simulink model "AirRefueling_Platform_PBVS_origin"  (R2022b)
settings: Solver=ode4  StartTime=0.0  StopTime=70  FixedStep=0.02  RelTol=1e-5  AbsTol=1e-4  EnableMultiTasking=on
InitFcn:
  | F16_Init
values from neighbouring files (symbols this model uses):
  airSpeed = 393.720000000000    (= 393.72)    [F16_Init.m]    (also in Initialization.m)
  alpha0 = trimAlpha*180/pi    (= 6.62393794015)    [F16_Init.m]    (also in Initialization.m)
  altitude = 9843    [F16_Init.m]    (also in Initialization.m)
  b_ref = 30.0    (= 30)    [F16_Init.m]    (also in Initialization.m)
  C = [ 1,0,0,zeros(1,15) ... (first row only)    [F16_Init.m]    (also in Initialization.m = [1,0,0,zeros(1,15))
  C2m = [C(1,:) ... (first row only)    [F16_Init.m]    (also in Initialization.m)
  d_f_rc = [3.75;0;-0.86]    [F16_Init.m]
  d_pr_rc = [6.06;0.54;-0.86]    [F16_Init.m]
  DeltaP = [0,0,DeltaP_z(j)]    [PBVS_main.m]
  dLEF = 0    [F16_Init.m]    (also in Initialization.m)
  fi_flag = 1    [F16_Init.m]    (also in Initialization.m)
  Kc = [ ... (first row only)    [F16_Init.m]    (also in Initialization.m)
  Ki = zeros(4,3)    [F16_Init.m]    (also in Initialization.m)
  Kp = zeros(4,18)    [F16_Init.m]    (also in Initialization.m)
  mass = 636.94    [F16_Init.m]    (also in Initialization.m)
  p0_rc = [-14.35-6.06-6;-0.54-(2);5.12+0.86-(-2)]    [F16_Init.m]
  q = zeros(N,1)    [hose3D_n_air_Fv_correction.m]
  trim_ail = 0.00874607850103852    (= 0.00874607850104)    [F16_Init.m]    (also in Initialization.m)
  trim_control = [trim_thrust;trim_ele;trim_ail;trim_rud]    [F16_Init.m]    (also in Initialization.m)
  trim_ele = -2.97973164860638    (= -2.97973164861)    [F16_Init.m]    (also in Initialization.m)
  trim_rud = 0.0680302158182712    (= 0.0680302158183)    [F16_Init.m]    (also in Initialization.m)
  trim_state1 = [trim_state;0;0;0;0;0;0]    [F16_Init.m]    (also in Initialization.m)
  trim_thrust = 2279.08519954656    (= 2279.08519955)    [F16_Init.m]    (also in Initialization.m)
undefined symbols (not defined in the file or in its folder): F, gray, MIL, vt0
libraries: aerolibconvert2 x6, aerolibasang x4, aerolibwind2 x2, aerolibobsolete x2, visionmorphops x2, vrlib x1, simulink x1, aerolibatmos2 x1, aerolibadyn x1, aerolibanimutils x1
(part 1 of 2)
settings Model: Creator=WhisPer  LastModifiedBy=Jinrui
settings SolverCC: AutoScaleAbsTol=off  AlgebraicLoopSolver=TrustRegion
settings DataIOCC: LimitDataPoints=on  SaveFormat=Array  ReturnWorkspaceOutputs=off
settings OptimizationCC: LifeSpan=inf
settings DebuggingCC: UnderspecifiedInitializationDetection=Classic  MergeDetectMultiDrivingBlocksExec=none  SolverPrmCheckMsg=warning  UnconnectedInputMsg=warning  UnconnectedOutputMsg=warning  UnconnectedLineMsg=warning  StateNameClashWarn=warning  SFUnexpectedBacktrackingDiag=warning  SFNoUnconditionalDefaultTransitionDiag=warning  SFExecutionAtInitializationDiag=none  SFMachineParentedDataDiag=warning  ArithmeticOperatorsInVariantConditions=warning
settings HardwareCC: ProdBitPerPointer=32  ProdBitPerSizeT=32  ProdBitPerPtrDiffT=32  ProdLargestAtomicFloat=None  ProdIntDivRoundTo=Undefined  ProdEndianess=Unspecified  ProdWordSize=32  ProdHWDeviceType=32-bit Generic
settings ModelReferenceCC: EnableRefExpFcnMdlSchedulingChecks=on  PropagateSignalLabelsOutOfModel=off
settings SFSimCC: SimUseLocalCustomCode=off  CustomCodeUndefinedFunction=UseInterfaceOnly
settings RTWCC: RTWUseLocalCustomCode=off
settings CodeAppCC: StateflowObjectComments=on
settings GRTTargetCC: TargetLangStandard=C89/C90 (ANSI)
settings ConfigComp: CovMetricSettings=dw  CovSaveCumulativeToWorkspaceVar=on  CovSaveSingleToWorkspaceVar=on  CovExternalEMLEnable=off

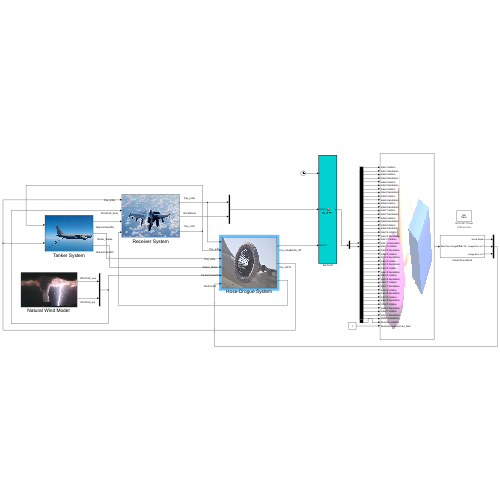
[thumbnail: Simulink's stored preview of the top-level diagram]
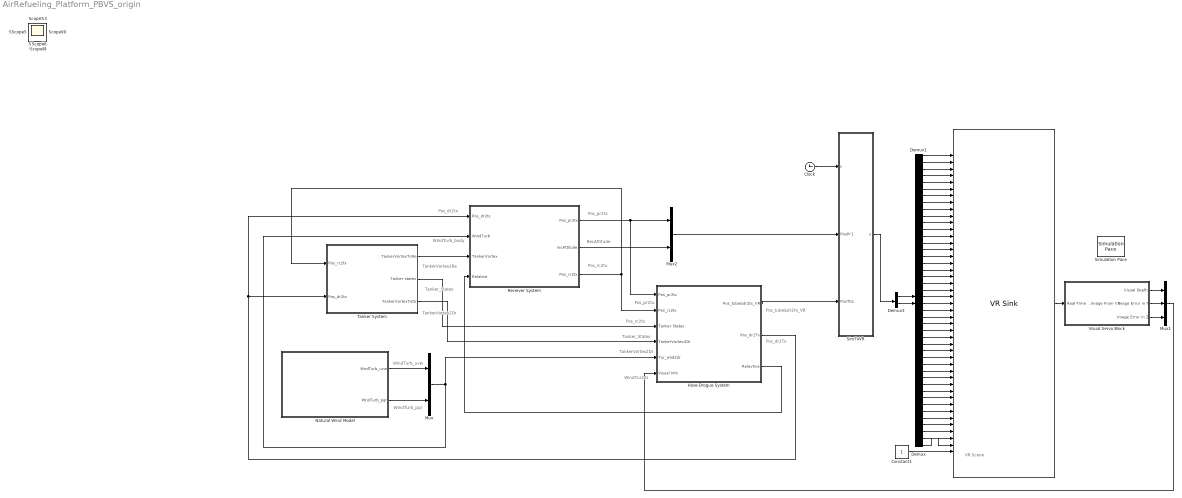
== system AirRefueling_Platform_PBVS_origin ==
  note: Pos_pr2tx
  note: RecAttitude
  note: WindTurb_uvw
  note: WindTurb_pqr
  note: Pos_dr2Tx
  note: Pos_tube&dr2tx_VR
  note: WindTur2dr
  note: Pos_pr2tx
  note: WindTurb_body
  note: Pos_dr2tx
  note: Pos_rc2tx
  note: TankerVortex2Re
  note: TankerVortex2Dr
  note: Tanker_States
  note: Tanker_States
  note: TankerVortex2Dr
  note: Pos_rc2tx
  note: VR Scene
  " " : vrlib/VR Sink  InstantiateOnLoad=on  SampleTime=-1  ViewEnable=on  RemoteChange=off  RemoteView=off  FieldsWritten=tube1.rotation.4.1.1.double#tube1.translation.3.1.1.double#tube2.rotation.4.1.1.double#tube2.translation.3.1.1.double#tube3.rotation.4.1.1.double#tube3.translation.3.1.1.double#tube4.rotation.4.1.1.double#tube4.translation.3.1.1.double#tube5.rotation.4.1.1.double#tube5.translation.3.1.1.double#tube6.rotation.4.1.1.double#tube6.translation.3.1.1.double#tube7.rotation.4.1.1.double#tube7.translation.3.1.1.double#tube8.rotation.4.1.1.double#tube8.translation.3.1.1.double#tube9.rotation.4.1.1.double#tube9.translation.3.1.1.double#tube10.rotation.4.1.1.double#tube10.translation.3.1.1.double#tube11.rotation.4.1.1.double#tube11.translation.3.1.1.double#tube12.rotation.4.1.1.double#tube12.translation.3.1.1.double#tube13.rotation.4.1.1.double#tube13.translation.3.1.1.double#tube14.rotation.4.1.1.double#tube14.translation.3.1.1.double#tube15.rotation.4.1.1.double#tube15.translation.3.1.1.double#tube16.rotation.4.1.1.double#tube16.translation.3.1.1.double#tube17.rotation.4.1.1.double#tube17.translation.3.1.1.double#tube18.rotation.4.1.1.double#tube18.translation.3.1.1.double#tube19.rotation.4.1.1.double#tube19.translation.3.1.1.double#tube20.rotation.4.1.1.double#tube20.translation.3.1.1.double#tube21.rotation.4.1.1.double#tube21.translation.3.1.1.double#ASDD.translation.3.1.1.double#Receiver.rotation.4.1.1.double#ReceiverViewPoint.set_bind.1.1.1.logical  WorldFileName=AirRefuelingTubeSim_Image.WRL  AutoView=off  VideoDimensions=[200 320]  AllowVariableSize=off  FigureProperties="{'Position', 'Name', 'Viewpoint', 'CameraBound', 'CameraDirection', 'CameraPosition', 'CameraUpVector', 'ZoomFactor', 'Antialiasing', 'Headlight', 'Lighting', 'NavPanel', 'Sound', 'StatusBar', 'Stereo3D', 'Stereo3DCameraOffset', 'Stereo3DHIT', 'ToolBar', 'Textures', 'Transparency', 'Triad', 'Wireframe', 'NavZones', 'NavMode', 'NavSpeed', 'CaptureFileFormat', 'CaptureFileName', 'Record2DCompressMethod', 'Record2DCompressQuality', 'Record2D', 'Record2DFileName', 'Record2DFPS'; [3.0000000000000000e+01   6.0000000000000000e+01   3.2000000000000000e+02   2.0000000000000000e+02], '', 'Receive1', 'on', [0.0000000000000000e+00   0.0000000000000000e+00  -1.0000000000000000e+00], [0.0000000000000000e+00   0.0000000000000000e+00   0.0000000000000000e+00], [0.0000000000000000e+00   1.0000000000000000e+00   0.0000000000000000e+00], [1.0000000000000000e+00], 'on', 'on', 'on', 'none', 'on', 'off', 'off', [1.0000000149011612e-01], [0.0000000000000000e+00], 'off', 'on', 'on', 'none', 'off', 'off', 'walk', 'normal', 'tif', '%f_anim_%n.tif', 'auto', [7.5000000000000000e+01], 'off', '***video***', 'auto'}"
  Clock : Clock
  Constant1 : Constant
  Demux : Demux  Outputs=22
  Demux1 : Demux  Outputs=22
  Demux3 : Demux  Outputs=[88,66]
  Hose-Drogue System : Subsystem
      mask Display: image(imread('Icon\drogue.jpg'))
  Mux : Mux  Inputs=2
  Mux1 : Mux  Inputs=3
  Mux2 : Mux  Inputs=2
  "Natural Wind Model " : Subsystem
      mask Display: image(imread('Icon\Enviroment.jpg'))
  Receiver System : Subsystem
      mask Display: image(imread('Icon\f16thumb.jpg'))
  SimToVR : MATLAB Function  TreatAsAtomicUnit=on
  Simulation Pace : aerolibanimutils/Simulation Pace  SimulationPace=1000  SleepMode=MATLAB Thread  OutputPaceError=off  SampleTime=-1
  Tanker System : Subsystem
      mask Display: image(imread('Icon\tanker.jpg'))
  Visual Servo Block : Subsystem
      mask Display: image('icon/camera.jpg');
  Scope{,1,3..34} (34 alike) : Scope
  wires:
  Receiver System/1(Pos_pr2tx) -> Hose-Drogue System/1(Pos_pr2tx), Mux2/1
  Hose-Drogue System/2(Pos_dr2Tx) -> Tanker System/2(Pos_dr2tx), Receiver System/1(Pos_dr2tx)
  Mux/1 -> Receiver System/2(WindTurb), Hose-Drogue System/5(Tur_wnd2dr)
  Receiver System/2(recAttitude) -> Mux2/2
  "Natural Wind Model "/1(WndTurb_uvw) -> Mux/1
  "Natural Wind Model "/2(WndTurb_pqr) -> Mux/2
  Tanker System/2(Tanker states) -> Hose-Drogue System/3(Tanker States)
  Tanker System/3(TankerVortexToDr) -> Hose-Drogue System/4(TankerVortex2Dr)
  Tanker System/1(TankerVortexToRe) -> Receiver System/3(TankerVortex)
  Receiver System/3(Pos_rc2tx) -> Hose-Drogue System/2(Pos_rc2tx), Tanker System/1(Pos_rc2tx)
  Hose-Drogue System/3(Relavtive) -> Receiver System/4(Relative)
  Hose-Drogue System/1(Pos_tube&dr2tx_VR) -> SimToVR/3(PosTb1)
  Mux2/1 -> SimToVR/2(PosPr1)
  Demux3/2 -> Demux/1
  Demux/22 -> " "/43
  Demux1/22 -> " "/44
  Demux3/1 -> Demux1/1
  Clock/1 -> SimToVR/1(t)
  Demux1/1 -> " "/1
  Demux/1 -> " "/2
  Demux1/2 -> " "/3
  Demux/2 -> " "/4
  Demux1/3 -> " "/5
  Demux/3 -> " "/6
  Demux1/4 -> " "/7
  Demux/4 -> " "/8
  Demux1/5 -> " "/9
  Demux/5 -> " "/10
  Demux1/6 -> " "/11
  Demux/6 -> " "/12
  Demux1/7 -> " "/13
  Demux/7 -> " "/14
  Demux1/8 -> " "/15
  Demux/8 -> " "/16
  Demux1/9 -> " "/17
  Demux/9 -> " "/18
  Demux1/10 -> " "/19
  Demux/10 -> " "/20
  Demux1/11 -> " "/21
  Demux/11 -> " "/22
  Demux1/12 -> " "/23
  Demux/12 -> " "/24
  Demux1/13 -> " "/25
  Demux/13 -> " "/26
  Demux1/14 -> " "/27
  Demux/14 -> " "/28
  Demux1/15 -> " "/29
  Demux/15 -> " "/30
  Demux1/16 -> " "/31
  Demux/16 -> " "/32
  Demux1/17 -> " "/33
  Demux/17 -> " "/34
  Demux1/18 -> " "/35
  Demux/18 -> " "/36
  Demux1/19 -> " "/37
  Demux/19 -> " "/38
  Demux1/20 -> " "/39
  Demux/20 -> " "/40
  Demux1/21 -> " "/41
  Demux/21 -> " "/42
  Constant1/1 -> " "/45
  " "/1 -> Visual Servo Block/1(Real-Time Image From VR)
  Visual Servo Block/1(Visual Depth) -> Mux1/1
  Visual Servo Block/2(Image Error in Y) -> Mux1/2
  Visual Servo Block/3(Image Error in Z) -> Mux1/3
  SimToVR/1(y) -> Demux3/1
  Mux1/1 -> Hose-Drogue System/6(Visual Info)

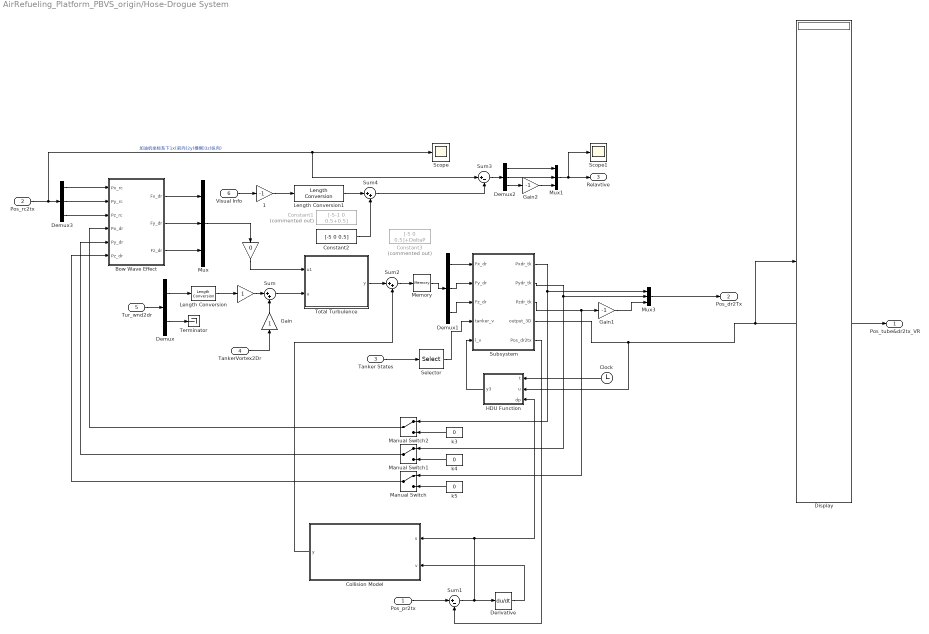
== system AirRefueling_Platform_PBVS_origin/Hose-Drogue System ==
  Pos_pr2tx : Inport
  Pos_rc2tx : Inport  Port=2
  Tanker States : Inport  Port=3
  TankerVortex2Dr : Inport  Port=4
  Tur_wnd2dr : Inport  Port=5
  Visual Info : Inport  Port=6
  " " : Gain
  "  " : Gain  Gain=0
  "  1" : Gain  Gain=-1
  Bow Wave Effect : Subsystem
  Clock : Clock
  Collision Model : MATLAB Function  TreatAsAtomicUnit=on
  Constant1 : Constant  Commented=on  Value=[-5-1 0 0.5+0.5]
  Constant2 : Constant  Value=[-5 0 0.5]
  Constant3 : Constant  Commented=on  Value=[-5 0 0.5]+DeltaP
  Demux : Demux  Outputs=2
  Demux1 : Demux  Outputs=3
  Demux2 : Demux  Outputs=3
  Demux3 : Demux  Outputs=3
  Derivative : Derivative
  Display : Display
  Gain : Gain
  Gain1 : Gain  Gain=-1
  Gain2 : Gain  Gain=-1
  HDU Function : MATLAB Function  TreatAsAtomicUnit=on
  Length Conversion : aerolibconvert2/Length Conversion  IU=ft  OU=m
  Length Conversion1 : aerolibconvert2/Length Conversion  IU=ft  OU=m
  Manual Switch : ManualSwitch
  Manual Switch1 : ManualSwitch
  Manual Switch2 : ManualSwitch
  Memory : Memory
  Mux : Mux  Inputs=3
  Mux1 : Mux  Inputs=3
  Mux3 : Mux  Inputs=3
  Scope : Scope
  Scope1 : Scope
  Selector : Selector  InputPortWidth=9  IndexOptions=Index vector (dialog)  Indices=[4 5 6]  OutputSizes=1
  Subsystem : Subsystem
  Sum : Sum  Inputs=|++
  Sum1 : Sum  Inputs=|+-
  Sum2 : Sum  Inputs=|++
  Sum3 : Sum  Inputs=|+-
  Sum4 : Sum  Inputs=|++
  Terminator : Terminator
  "Total Turbulence  " : MATLAB Function  TreatAsAtomicUnit=on
  k3 : Constant  Value=0
  k4 : Constant  Value=0
  k5 : Constant  Value=0
  Pos_tube&dr2tx_VR : Outport
  Pos_dr2Tx : Outport  Port=2
  Relavtive : Outport  Port=3
  wires:
  Mux/1 -> "  "/1
  TankerVortex2Dr/1 -> Gain/1
  Demux/1 -> Length Conversion/1
  Demux1/3 -> Subsystem/3(Fz_dr)
  Demux1/2 -> Subsystem/2(Fy_dr)
  Demux1/1 -> Subsystem/1(Fx_dr)
  Demux/2 -> Terminator/1
  Tur_wnd2dr/1 -> Demux/1
  Pos_rc2tx/1 -> Sum3/1, Scope/1, Demux3/1  "加油机坐标系下1x(前向)2y(横侧)3z(纵向)"
  Bow Wave Effect/3(Fz_dr) -> Mux/3
  Sum/1 -> "Total Turbulence  "/2(u)
  Bow Wave Effect/2(Fy_dr) -> Mux/2
  Bow Wave Effect/1(Fx_dr) -> Mux/1
  Demux3/1 -> Bow Wave Effect/1(Px_rc)
  k4/1 -> Manual Switch1/2
  Manual Switch1/1 -> Bow Wave Effect/5(Py_dr)
  Manual Switch2/1 -> Bow Wave Effect/4(Px_dr)
  k5/1 -> Manual Switch/2
  k3/1 -> Manual Switch2/2
  Mux3/1 -> Pos_dr2Tx/1
  Manual Switch/1 -> Bow Wave Effect/6(Pz_dr)
  Subsystem/2(Pydr_tk) -> Manual Switch1/1, Mux3/2
  Subsystem/1(Pxdr_tk) -> Manual Switch2/1, Mux3/1
  Gain1/1 -> Mux3/3
  Subsystem/3(Pzdr_tk) -> Gain1/1, Manual Switch/1
  Demux3/3 -> Bow Wave Effect/3(Pz_rc)
  Demux3/2 -> Bow Wave Effect/2(Py_rc)
  "Total Turbulence  "/1(y) -> Sum2/1
  Subsystem/4(output_3D) -> Display/1, Pos_tube&dr2tx_VR/1, HDU Function/2(u)
  Gain/1 -> Sum/2
  " "/1 -> Sum/1
  "  "/1 -> "Total Turbulence  "/1(u1)
  Length Conversion/1 -> " "/1
  Tanker States/1 -> Selector/1
  Sum1/1 -> Collision Model/1(u), HDU Function/3(dp), Derivative/1
  Derivative/1 -> Collision Model/2(v)
  Sum2/1 -> Memory/1
  Selector/1 -> Subsystem/4(tanker_v)
  Subsystem/5(Pos_dr2tx) -> Sum1/2
  Memory/1 -> Demux1/1
  Clock/1 -> HDU Function/1(t)
  HDU Function/1(y3) -> Subsystem/5(l_v)
  Pos_pr2tx/1 -> Sum1/1
  Visual Info/1 -> "  1"/1
  "  1"/1 -> Length Conversion1/1
  Length Conversion1/1 -> Sum4/1
  Sum4/1 -> Sum3/2
  Constant2/1 -> Sum4/2
  Demux2/2 -> Mux1/2
  Demux2/1 -> Mux1/1
  Gain2/1 -> Mux1/3
  Demux2/3 -> Gain2/1
  Mux1/1 -> Relavtive/1, Scope1/1
  Sum3/1 -> Demux2/1
  Collision Model/1(y) -> Sum2/2

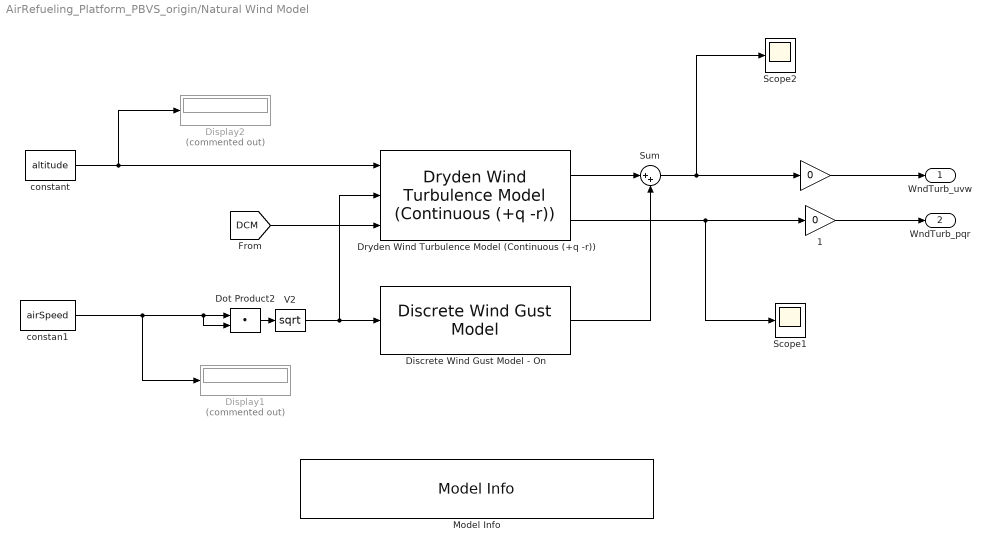
== system AirRefueling_Platform_PBVS_origin/Natural Wind Model  ==
  " " : Gain  Gain=0
  " 1" : Gain  Gain=0
  Discrete Wind Gust Model - On : aerolibwind2/Discrete Wind Gust Model  units=English (Velocity in ft/s)  Gx=on  Gy=on  Gz=on  t_0=20  d_m=[120 120 80]  v_m=[0 0 0]
  Display1 : Display  Commented=on
  Display2 : Display  Commented=on
  Dot Product2 : DotProduct  SaturateOnIntegerOverflow=on  InputSameDT=off  OutDataTypeStr=Inherit: Inherit via internal rule
  Dryden Wind Turbulence Model (Continuous (+q -r)) : aerolibwind2/Dryden Wind Turbulence Model  (Continuous (+q -r))  units=English (Velocity in ft/s)  spec=MIL-F-8785C  model=Continuous Dryden (+q -r)  W20=5  Wdeg=0  TurbProb=2x10^-1  L_high=533.5  Wingspan=6  ts=0.02  Seed=1+fix(3650*rand(1,4))  T_on=on
  Model Info : simulink/Model-Wide Utilities/Model Info  Frame=on  DisplayStringWithTags=|  HorizontalTextAlignment=Center  LeftAlignmentValue=0.5
      | The resultant mean wind speed and angular rates is in the body-fixed axis. 
      | The simulation parameter is set to
      | altitude:3000m
      | airspeed:120m/s
  Scope1 : Scope
  Scope2 : Scope
  Sum : Sum  Inputs=|++  InputSameDT=on  SaturateOnIntegerOverflow=on  OutDataTypeStr=Inherit: Same as first input
  V2 : Math  Operator=sqrt  SignedPower=on
  constan1 : Constant  Value=airSpeed
  constant : Constant  Value=altitude
  WndTurb_uvw : Outport
  WndTurb_pqr : Outport  Port=2
  wires:
  [DCM] -> Dryden Wind Turbulence Model (Continuous (+q -r))/3
  V2/1 -> Dryden Wind Turbulence Model (Continuous (+q -r))/2, Discrete Wind Gust Model - On/1
  Dot Product2/1 -> V2/1
  constan1/1 -> Dot Product2/1, Dot Product2/2, Display1/1
  Discrete Wind Gust Model - On/1 -> Sum/2
  Dryden Wind Turbulence Model (Continuous (+q -r))/2 -> Scope1/1, " 1"/1
  Dryden Wind Turbulence Model (Continuous (+q -r))/1 -> Sum/1
  Sum/1 -> Scope2/1, " "/1
  constant/1 -> Display2/1, Dryden Wind Turbulence Model (Continuous (+q -r))/1
  " "/1 -> WndTurb_uvw/1
  " 1"/1 -> WndTurb_pqr/1

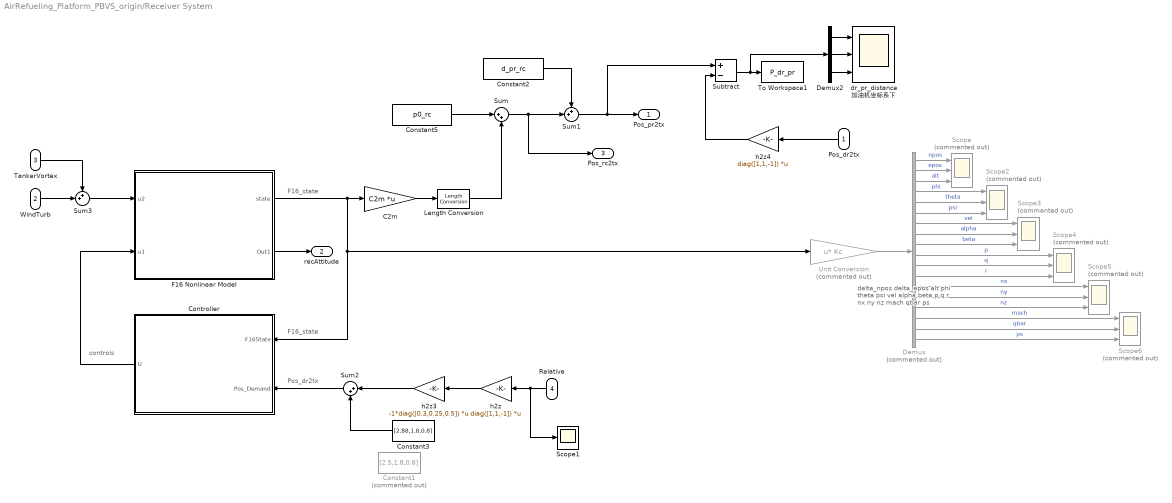
== system AirRefueling_Platform_PBVS_origin/Receiver System ==
  note: controls
  note: Pos_dr2tx
  note: F16_state
  note: delta_npos
      | delta_epos
      | alt
      | phi
      | theta
      | psi
      | vel
      | alpha
      | beta
      | p
      | q
      | r
      | nx
      | ny
      | nz
      | mach
      | qbar
      | ps
  note: F16_state
  Pos_dr2tx : Inport
  WindTurb : Inport  Port=2
  TankerVortex : Inport  Port=3
  Relative : Inport  Port=4
  C2m : Gain  Gain=C2m  Multiplication=Matrix(K*u) (u vector)
  Constant1 : Constant  Commented=on  Value=[2.5,1.8,0.8]
  Constant2 : Constant  Value=d_pr_rc
  Constant3 : Constant  Value=[2.88,1.8,0.8]
  Constant5 : Constant  Value=p0_rc
  Controller : Subsystem
      mask Display: image(imread('Icon\F16_Pilot.jpg'))
  Demux : Demux  Commented=on  Outputs=18
      settings: DisplayOption=none
  Demux2 : Demux  Outputs=3
  F16 Nonlinear Model : Subsystem
      mask Display: image(imread('Icon\fighter_f16.jpg'))
  Length Conversion : aerolibconvert2/Length Conversion  IU=ft  OU=m
  Scope{,2..6} (6 alike) : Scope  Commented=on  NumInputPorts=3
  Scope1 : Scope
  Subtract : Sum  Inputs=+-
  Sum : Sum  Inputs=|++
  Sum1 : Sum  Inputs=++|
  Sum2 : Sum  Inputs=|++
  Sum3 : Sum  Inputs=++|
  To Workspace1 : ToWorkspace  VariableName=P_dr_pr  SampleTime=-1
  Unit Conversion : Gain  Commented=on  Gain=Kc  Multiplication=Matrix(u*K)
  dr_pr_distance 加油机坐标系下 : Scope  NumInputPorts=3
  h2z : Gain  Gain=diag([1,1,-1])  Multiplication=Matrix(K*u)
  h2z3 : Gain  Gain=-1*diag([0.3,0.25,0.5])  Multiplication=Matrix(K*u)
  h2z4 : Gain  Gain=diag([1,1,-1])  Multiplication=Matrix(K*u)
  Pos_pr2tx : Outport
  recAttitude : Outport  Port=2
  Pos_rc2tx : Outport  Port=3
  wires:
  Controller/1(U) -> F16 Nonlinear Model/2(u1)
  WindTurb/1 -> Sum3/2
  F16 Nonlinear Model/1(state) -> C2m/1, Controller/1(F16State), Unit Conversion/1
  Demux/1 -> Scope/1  "npos"
  Demux/2 -> Scope/2  "epos"
  Demux/3 -> Scope/3  "alt"
  Demux/5 -> Scope2/2  "theta"
  Demux/6 -> Scope2/3  "psi"
  Demux/7 -> Scope3/1  "vel"
  Demux/8 -> Scope3/2  "alpha"
  Demux/9 -> Scope3/3  "beta"
  Demux/10 -> Scope4/1  "p"
  Demux/11 -> Scope4/2  "q"
  Demux/12 -> Scope4/3  "r"
  Demux/13 -> Scope5/1  "nx"
  Demux/14 -> Scope5/2  "ny"
  Demux/15 -> Scope5/3  "nz"
  Demux/4 -> Scope2/1  "phi"
  Demux/16 -> Scope6/1  "mach"
  Demux/17 -> Scope6/2  "qbar"
  Demux/18 -> Scope6/3  "ps"
  Unit Conversion/1 -> Demux/1
  F16 Nonlinear Model/2(Out1) -> recAttitude/1
  C2m/1 -> Length Conversion/1
  Sum3/1 -> F16 Nonlinear Model/1(u2)
  TankerVortex/1 -> Sum3/1
  Length Conversion/1 -> Sum/2
  Constant5/1 -> Sum/1
  Sum1/1 -> Pos_pr2tx/1, Subtract/1
  Sum/1 -> Pos_rc2tx/1, Sum1/2
  Constant2/1 -> Sum1/1
  h2z/1 -> h2z3/1
  Sum2/1 -> Controller/2(Pos_Demand)
  h2z3/1 -> Sum2/1
  Constant3/1 -> Sum2/2
  Pos_dr2tx/1 -> h2z4/1
  Subtract/1 -> Demux2/1, To Workspace1/1
  Demux2/2 -> dr_pr_distance 加油机坐标系下/2
  Demux2/1 -> dr_pr_distance 加油机坐标系下/1
  Demux2/3 -> dr_pr_distance 加油机坐标系下/3
  h2z4/1 -> Subtract/2
  Relative/1 -> Scope1/1, h2z/1

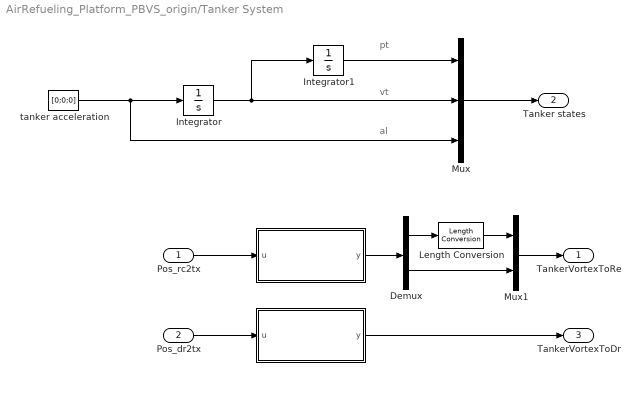
== system AirRefueling_Platform_PBVS_origin/Tanker System ==
  note: pt
  note: vt
  note: al
  Pos_rc2tx : Inport
  Pos_dr2tx : Inport  Port=2
  " " : MATLAB Function  TreatAsAtomicUnit=on
  "  " : MATLAB Function  TreatAsAtomicUnit=on
  Demux : Demux  Outputs=2
  Integrator : Integrator  InitialCondition=vt0
  Integrator1 : Integrator  InitialCondition=[0;0;0]
  Length Conversion : aerolibconvert2/Length Conversion  IU=m  OU=ft
  Mux : Mux  Inputs=3
  Mux1 : Mux  Inputs=2
  tanker acceleration : Constant  Value=[0;0;0]
  TankerVortexToRe : Outport
  Tanker states : Outport  Port=2
  TankerVortexToDr : Outport  Port=3
  wires:
  tanker acceleration/1 -> Mux/3, Integrator/1
  Integrator/1 -> Mux/2, Integrator1/1
  Mux/1 -> Tanker states/1
  Pos_rc2tx/1 -> " "/1(u)
  Pos_dr2tx/1 -> "  "/1(u)
  "  "/1(y) -> TankerVortexToDr/1
  Integrator1/1 -> Mux/1
  " "/1(y) -> Demux/1
  Mux1/1 -> TankerVortexToRe/1
  Demux/2 -> Mux1/2
  Length Conversion/1 -> Mux1/1
  Demux/1 -> Length Conversion/1

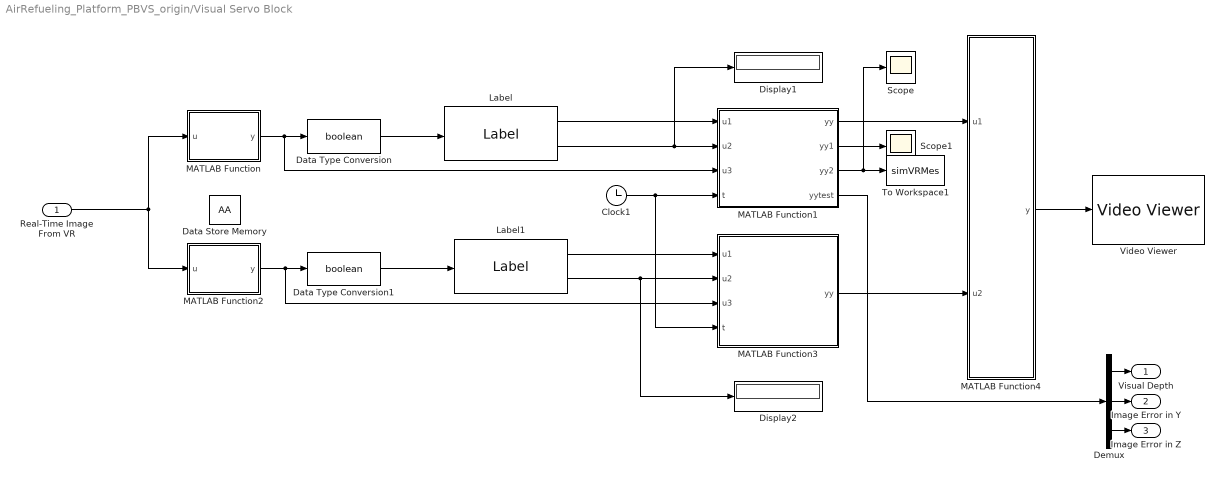
== system AirRefueling_Platform_PBVS_origin/Visual Servo Block ==
  Real-Time Image From VR : Inport
  Clock1 : Clock
  Data Store Memory : DataStoreMemory  DataStoreName=AA  InitialValue=[0 0 0]  ShowAdditionalParam=off  OutDataTypeStr=double
  Data Type Conversion : DataTypeConversion  OutDataTypeStr=boolean  SaturateOnIntegerOverflow=off  RndMeth=Floor
  Data Type Conversion1 : DataTypeConversion  OutDataTypeStr=boolean  SaturateOnIntegerOverflow=off  RndMeth=Floor
  Demux : Demux  Outputs=3
  Display1 : Display
  Display2 : Display
  Label : visionmorphops/Label  conn=8  output=Label matrix and number of labels  outType=Automatic  lastLabel=maximum value of the output data type
  Label1 : visionmorphops/Label  conn=8  output=Label matrix and number of labels  outType=Automatic  lastLabel=maximum value of the output data type
  MATLAB Function : MATLAB Function  TreatAsAtomicUnit=on
  MATLAB Function1 : MATLAB Function  TreatAsAtomicUnit=on
  MATLAB Function2 : MATLAB Function  TreatAsAtomicUnit=on
  MATLAB Function3 : MATLAB Function  TreatAsAtomicUnit=on
  MATLAB Function4 : MATLAB Function  TreatAsAtomicUnit=on
  Scope : Scope
  Scope1 : Scope
  To Workspace1 : ToWorkspace  VariableName=simVRMes  SampleTime=-1
  Video Viewer : VideoViewer  colormapValue=gray(256)  FigPos=[840 825 710 515]
  Visual Depth : Outport
  Image Error in Y : Outport  Port=2
  Image Error in Z : Outport  Port=3
  wires:
  Real-Time Image From VR/1 -> MATLAB Function/1(u), MATLAB Function2/1(u)
  Label/1 -> MATLAB Function1/1(u1)
  MATLAB Function/1(y) -> MATLAB Function1/3(u3), Data Type Conversion/1
  Data Type Conversion/1 -> Label/1
  MATLAB Function2/1(y) -> MATLAB Function3/3(u3), Data Type Conversion1/1
  Data Type Conversion1/1 -> Label1/1
  Label1/1 -> MATLAB Function3/1(u1)
  Label1/2 -> Display2/1, MATLAB Function3/2(u2)
  MATLAB Function1/1(yy) -> MATLAB Function4/1(u1)
  MATLAB Function3/1(yy) -> MATLAB Function4/2(u2)
  MATLAB Function4/1(y) -> Video Viewer/1
  Clock1/1 -> MATLAB Function3/4(t), MATLAB Function1/4(t)
  Label/2 -> Display1/1, MATLAB Function1/2(u2)
  MATLAB Function1/4(yytest) -> Demux/1
  Demux/1 -> Visual Depth/1
  Demux/2 -> Image Error in Y/1
  Demux/3 -> Image Error in Z/1
  MATLAB Function1/3(yy2) -> Scope/1, To Workspace1/1
  MATLAB Function1/2(yy1) -> Scope1/1

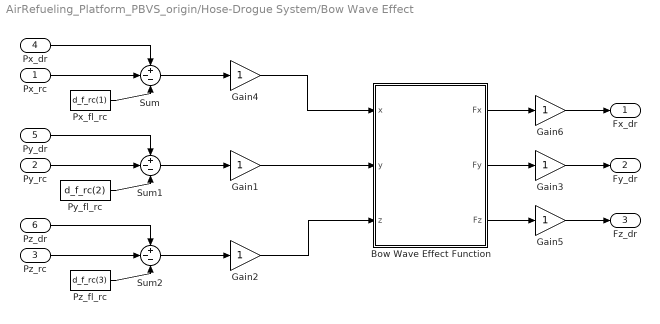
== system AirRefueling_Platform_PBVS_origin/Hose-Drogue System/Bow Wave Effect ==
  Px_rc : Inport
  Py_rc : Inport  Port=2
  Pz_rc : Inport  Port=3
  Px_dr : Inport  Port=4
  Py_dr : Inport  Port=5
  Pz_dr : Inport  Port=6
  Bow Wave Effect Function : MATLAB Function  TreatAsAtomicUnit=on
  Gain{1..6} (6 alike) : Gain
  Px_fl_rc : Constant  Value=d_f_rc(1)
  Py_fl_rc : Constant  Value=d_f_rc(2)
  Pz_fl_rc : Constant  Value=d_f_rc(3)
  Sum : Sum  Inputs=+--
  Sum1 : Sum  Inputs=+--
  Sum2 : Sum  Inputs=+--
  Fx_dr : Outport
  Fy_dr : Outport  Port=2
  Fz_dr : Outport  Port=3
  wires:
  Sum2/1 -> Gain2/1
  Sum1/1 -> Gain1/1
  Bow Wave Effect Function/3(Fz) -> Gain5/1
  Bow Wave Effect Function/2(Fy) -> Gain3/1
  Bow Wave Effect Function/1(Fx) -> Gain6/1
  Gain6/1 -> Fx_dr/1
  Gain5/1 -> Fz_dr/1
  Gain3/1 -> Fy_dr/1
  Gain2/1 -> Bow Wave Effect Function/3(z)
  Gain1/1 -> Bow Wave Effect Function/2(y)
  Gain4/1 -> Bow Wave Effect Function/1(x)
  Pz_dr/1 -> Sum2/1
  Pz_fl_rc/1 -> Sum2/3
  Pz_rc/1 -> Sum2/2
  Py_fl_rc/1 -> Sum1/3
  Py_dr/1 -> Sum1/1
  Py_rc/1 -> Sum1/2
  Px_dr/1 -> Sum/1
  Px_fl_rc/1 -> Sum/3
  Px_rc/1 -> Sum/2
  Sum/1 -> Gain4/1

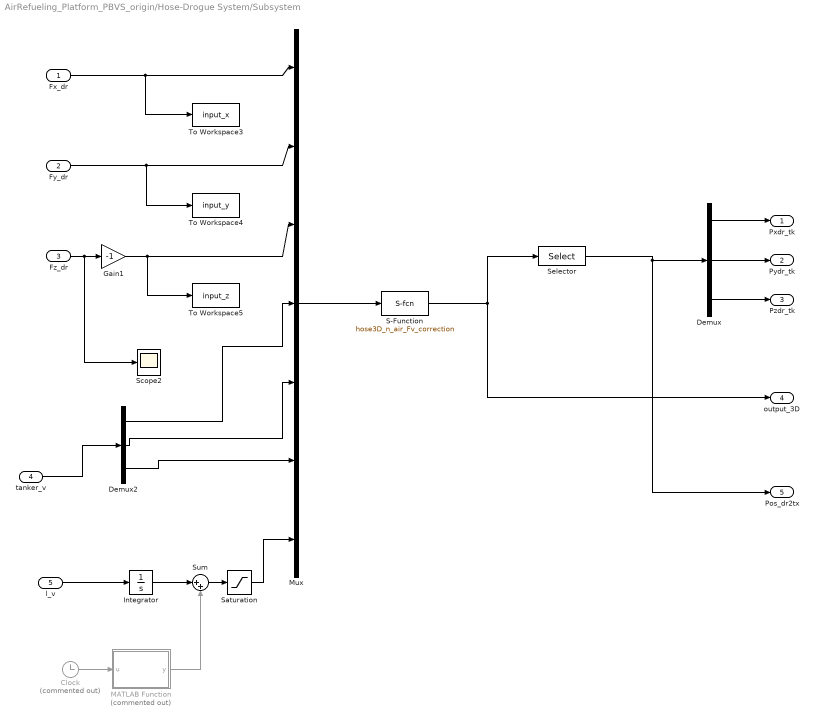
== system AirRefueling_Platform_PBVS_origin/Hose-Drogue System/Subsystem ==
  Fx_dr : Inport
  Fy_dr : Inport  Port=2
  Fz_dr : Inport  Port=3
  tanker_v : Inport  Port=4
  l_v : Inport  Port=5
  Clock : Clock  Commented=on
  Demux : Demux  Outputs=3
  Demux2 : Demux  Outputs=3
  Gain1 : Gain  Gain=-1  ParamDataTypeStr=double  OutDataTypeStr=double
  Integrator : Integrator
  MATLAB Function : MATLAB Function  Commented=on  TreatAsAtomicUnit=on
  Mux : Mux  Inputs=7
  S-Function : S-Function  FunctionName=hose3D_n_air_Fv_correction  SFunctionDeploymentMode=off  EnableBusSupport=off
  Saturation : Saturate  UpperLimit=13  LowerLimit=-1
  Scope2 : Scope
  Selector : Selector  InputPortWidth=100  IndexOptions=Index vector (dialog)  Indices=[58 59 60]  OutputSizes=1
  Sum : Sum  Inputs=|++
  To Workspace3 : ToWorkspace  VariableName=input_x  SampleTime=-1
  To Workspace4 : ToWorkspace  VariableName=input_y  SampleTime=-1
  To Workspace5 : ToWorkspace  VariableName=input_z  SampleTime=-1
  Pxdr_tk : Outport
  Pydr_tk : Outport  Port=2
  Pzdr_tk : Outport  Port=3
  output_3D : Outport  Port=4
  Pos_dr2tx : Outport  Port=5
  wires:
  Mux/1 -> S-Function/1
  Demux2/1 -> Mux/4
  Demux2/2 -> Mux/5
  Demux2/3 -> Mux/6
  Fy_dr/1 -> Mux/2, To Workspace4/1
  Fz_dr/1 -> Scope2/1, Gain1/1
  Fx_dr/1 -> To Workspace3/1, Mux/1
  Demux/1 -> Pxdr_tk/1
  Demux/2 -> Pydr_tk/1
  Demux/3 -> Pzdr_tk/1
  Gain1/1 -> Mux/3, To Workspace5/1
  S-Function/1 -> Selector/1, output_3D/1
  l_v/1 -> Integrator/1
  Sum/1 -> Saturation/1
  Integrator/1 -> Sum/1
  Clock/1 -> MATLAB Function/1(u)
  MATLAB Function/1(y) -> Sum/2
  Saturation/1 -> Mux/7
  tanker_v/1 -> Demux2/1
  Selector/1 -> Pos_dr2tx/1, Demux/1

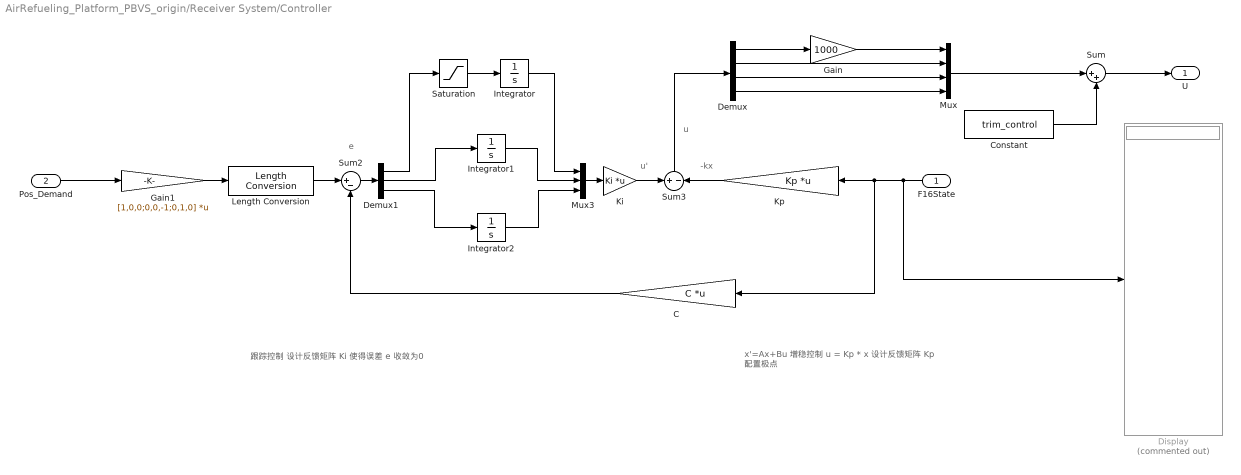
== system AirRefueling_Platform_PBVS_origin/Receiver System/Controller ==
  note: u
  note: -kx
  note: u'
  note: e
  note: 跟踪控制
      | 设计反馈矩阵 Ki 使得误差 e 收敛为0
  note: x'=Ax+Bu
      | 增稳控制 u = Kp * x
      | 设计反馈矩阵 Kp 配置极点
  F16State : Inport
  Pos_Demand : Inport  Port=2
  C : Gain  Gain=C  Multiplication=Matrix(K*u) (u vector)
  Constant : Constant  Value=trim_control
  Demux : Demux
  Demux1 : Demux  Outputs=3
  Display : Display  Commented=on
  Gain : Gain  Gain=1000
  Gain1 : Gain  Gain=[1,0,0;0,0,-1;0,1,0]  Multiplication=Matrix(K*u) (u vector)
  Integrator : Integrator
  Integrator1 : Integrator
  Integrator2 : Integrator
  Ki : Gain  Gain=Ki  Multiplication=Matrix(K*u) (u vector)
  Kp : Gain  Gain=Kp  Multiplication=Matrix(K*u) (u vector)
  Length Conversion : aerolibconvert2/Length Conversion  IU=m  OU=ft
  Mux : Mux
  Mux3 : Mux  Inputs=3
  Saturation : Saturate  UpperLimit=15  LowerLimit=-15
  Sum : Sum  Inputs=|++
  Sum2 : Sum  Inputs=|+-
  Sum3 : Sum  Inputs=+|-
  U : Outport
  wires:
  Sum2/1 -> Demux1/1
  C/1 -> Sum2/2
  Mux3/1 -> Ki/1
  Demux1/2 -> Integrator1/1
  F16State/1 -> Display/1, Kp/1, C/1
  Integrator1/1 -> Mux3/2
  Integrator/1 -> Mux3/1
  Demux1/3 -> Integrator2/1
  Integrator2/1 -> Mux3/3
  Length Conversion/1 -> Sum2/1
  Demux1/1 -> Saturation/1
  Ki/1 -> Sum3/1
  Kp/1 -> Sum3/2
  Sum3/1 -> Demux/1
  Saturation/1 -> Integrator/1
  Demux/2 -> Mux/2
  Demux/3 -> Mux/3
  Demux/4 -> Mux/4
  Demux/1 -> Gain/1
  Gain/1 -> Mux/1
  Pos_Demand/1 -> Gain1/1
  Gain1/1 -> Length Conversion/1
  Constant/1 -> Sum/2
  Mux/1 -> Sum/1
  Sum/1 -> U/1

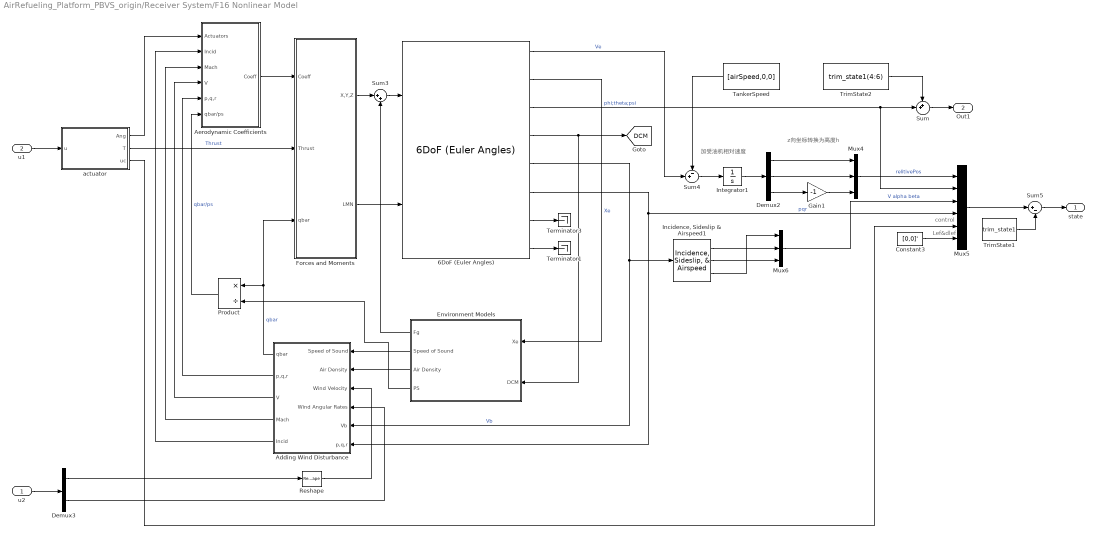
== system AirRefueling_Platform_PBVS_origin/Receiver System/F16 Nonlinear Model ==
  note: 加受油机相对速度
  note: z向坐标转换为高度h
  note: Lef&dlef
  note: control
  u2 : Inport
  u1 : Inport  Port=2
  6DoF (Euler Angles) : aerolibobsolete/6DoF (Euler Angles)  units=English (Velocity in ft/s)  mtype=Fixed  rep=Euler Angles  xme_0=xyz_0  Vm_0=uvw_0  eul_0=Euler_0  pm_0=pqr_0  mass_0=mass  mass_e=0.5  mass_f=2.0  inertia=Inertia  inertia_e=eye(3)  inertia_f=2*eye(3)  k_quat=1.0
  Adding Wind Disturbance : Subsystem
  Aerodynamic Coefficients : Subsystem
  Constant3 : Constant  Value=[0,0]'
  Demux2 : Demux  Outputs=3
  Demux3 : Demux  Outputs=2
  Environment Models : Subsystem
  Forces and Moments : Subsystem
  Gain1 : Gain  Gain=-1
  "Incidence, Sideslip & Airspeed1" : aerolibasang/Incidence, Sideslip, & Airspeed
  Integrator1 : Integrator
  Mux4 : Mux  Inputs=3
  Mux5 : Mux  Inputs=6
  Mux6 : Mux  Inputs=3
  Product : Product  Inputs=*/  InputSameDT=on  SaturateOnIntegerOverflow=on  OutDataTypeStr=Inherit: Same as first input
  Reshape : Reshape
  Sum : Sum  Inputs=++|
  Sum3 : Sum  Inputs=|++  InputSameDT=on  SaturateOnIntegerOverflow=on  OutDataTypeStr=Inherit: Same as first input
  Sum4 : Sum  Inputs=-+|
  Sum5 : Sum  Inputs=|+-
  TankerSpeed : Constant  Value=[airSpeed,0,0]
  Terminator1 : Terminator
  Terminator3 : Terminator
  TrimState1 : Constant  Value=trim_state1
  TrimState2 : Constant  Value=trim_state1(4:6)
  actuator : Subsystem
  state : Outport
  Out1 : Outport  Port=2
  tag scope: DCM=global
  wires:
  6DoF (Euler Angles)/8 -> Terminator1/1
  6DoF (Euler Angles)/7 -> Terminator3/1
  6DoF (Euler Angles)/4 -> Environment Models/2(DCM), [DCM]
  Adding Wind Disturbance/5(Incid) -> Aerodynamic Coefficients/2(Incid)
  Aerodynamic Coefficients/1(Coeff) -> Forces and Moments/1(Coeff)
  Environment Models/2(Speed of Sound) -> Adding Wind Disturbance/1(Speed of Sound)
  Environment Models/3(Air Density) -> Adding Wind Disturbance/2(Air Density)
  Forces and Moments/2(LMN) -> 6DoF (Euler Angles)/2
  Adding Wind Disturbance/1(qbar) -> Forces and Moments/3(qbar), Product/1  "qbar"
  Forces and Moments/1(X,Y,Z) -> Sum3/1
  Sum3/1 -> 6DoF (Euler Angles)/1
  Environment Models/1(Fg) -> Sum3/2
  Adding Wind Disturbance/3(V) -> Aerodynamic Coefficients/4(V)
  Adding Wind Disturbance/4(Mach) -> Aerodynamic Coefficients/3(Mach)
  Adding Wind Disturbance/2("p,q,r ") -> Aerodynamic Coefficients/5(p,q,r)
  Environment Models/4(PS) -> Product/2
  Product/1 -> Aerodynamic Coefficients/6(qbar/ps)  "qbar/ps"
  u1/1 -> actuator/1(u)
  actuator/2(T) -> Forces and Moments/2(Thrust)  "Thrust"
  actuator/1(Ang) -> Aerodynamic Coefficients/1(Actuators)
  6DoF (Euler Angles)/3 -> Mux5/2, Sum/2  "phi;theta;psi"
  "Incidence, Sideslip & Airspeed1"/1 -> Mux6/2
  "Incidence, Sideslip & Airspeed1"/2 -> Mux6/3
  Mux6/1 -> Mux5/3  "V alpha beta"
  "Incidence, Sideslip & Airspeed1"/3 -> Mux6/1
  6DoF (Euler Angles)/6 -> Adding Wind Disturbance/6(p,q,r), Mux5/4  "pqr"
  6DoF (Euler Angles)/5 -> Adding Wind Disturbance/5(Vb), "Incidence, Sideslip & Airspeed1"/1  "Vb"
  Mux5/1 -> Sum5/1
  TrimState1/1 -> Sum5/2
  Sum5/1 -> state/1
  actuator/3(uc) -> Mux5/5
  Constant3/1 -> Mux5/6
  Demux2/2 -> Mux4/2
  Demux2/3 -> Gain1/1
  Mux4/1 -> Mux5/1  "relitivePos"
  Demux2/1 -> Mux4/1
  Gain1/1 -> Mux4/3
  Sum4/1 -> Integrator1/1
  Integrator1/1 -> Demux2/1
  6DoF (Euler Angles)/2 -> Environment Models/1(Xe)  "Xe"
  u2/1 -> Demux3/1
  Reshape/1 -> Adding Wind Disturbance/3(Wind Velocity)
  Demux3/1 -> Reshape/1
  Sum/1 -> Out1/1
  Demux3/2 -> Adding Wind Disturbance/4(Wind Angular Rates)
  TrimState2/1 -> Sum/1
  6DoF (Euler Angles)/1 -> Sum4/2  "Ve"
  TankerSpeed/1 -> Sum4/1

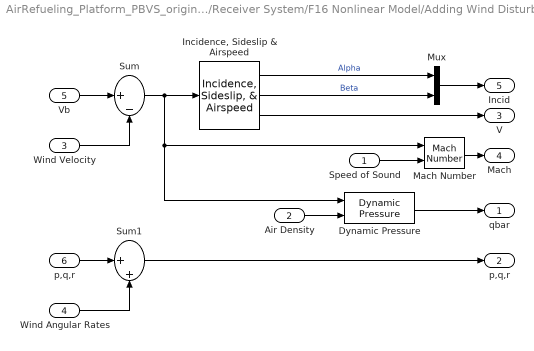
== system AirRefueling_Platform_PBVS_origin/Receiver System/F16 Nonlinear Model/Adding Wind Disturbance ==
  Speed of Sound : Inport
  Air Density : Inport  Port=2
  Wind Velocity : Inport  Port=3  PortDimensions=3
  Wind Angular Rates : Inport  Port=4  PortDimensions=3
  Vb : Inport  Port=5  PortDimensions=3
  p,q,r : Inport  Port=6  PortDimensions=3
  Dynamic Pressure : aerolibasang/Dynamic Pressure
  "Incidence, Sideslip & Airspeed" : aerolibasang/Incidence, Sideslip, & Airspeed
  Mach Number : aerolibasang/Mach Number
  Mux : Mux  Inputs=2
  Sum : Sum  Inputs=|+-  InputSameDT=on  SaturateOnIntegerOverflow=on  OutDataTypeStr=Inherit: Same as first input
  Sum1 : Sum  Inputs=|++  InputSameDT=on  SaturateOnIntegerOverflow=on  OutDataTypeStr=Inherit: Same as first input
  qbar : Outport  InitialOutput=0
  "p,q,r " : Outport  Port=2
  V : Outport  Port=3
  Mach : Outport  Port=4
  Incid : Outport  Port=5
  wires:
  "Incidence, Sideslip & Airspeed"/3 -> V/1
  Dynamic Pressure/1 -> qbar/1
  Air Density/1 -> Dynamic Pressure/2
  Mach Number/1 -> Mach/1
  Sum/1 -> Dynamic Pressure/1, Mach Number/1, "Incidence, Sideslip & Airspeed"/1
  Vb/1 -> Sum/1
  Speed of Sound/1 -> Mach Number/2
  Wind Velocity/1 -> Sum/2
  "Incidence, Sideslip & Airspeed"/2 -> Mux/2  "Beta"
  Mux/1 -> Incid/1
  "Incidence, Sideslip & Airspeed"/1 -> Mux/1  "Alpha"
  p,q,r/1 -> Sum1/1
  Wind Angular Rates/1 -> Sum1/2
  Sum1/1 -> "p,q,r "/1

== system AirRefueling_Platform_PBVS_origin/Receiver System/F16 Nonlinear Model/Aerodynamic Coefficients ==
  Actuators : Inport
  Incid : Inport  Port=2
  Mach : Inport  Port=3
  V : Inport  Port=4
  p,q,r : Inport  Port=5
  qbar/ps : Inport  Port=6
  Angle Conversion : aerolibconvert2/Angle Conversion  IU=rad  OU=deg
  Interpreted MATLAB Function : MATLABFcn  MATLABFcn=F16Coef1  OutputDimensions=6
  Leading Edge Flap : Subsystem
  Mux : Mux  Inputs=6
  Terminator2 : Terminator
  alpha : Selector  InputPortWidth=2  IndexOptions=Index vector (dialog)  Indices=1  OutputSizes=1
  flag : Constant  Value=fi_flag
  Coeff : Outport  InitialOutput=0
  wires:
  Angle Conversion/1 -> alpha/1, Mux/2
  Incid/1 -> Angle Conversion/1
  qbar/ps/1 -> Leading Edge Flap/2(qbar/ps)
  alpha/1 -> Leading Edge Flap/1(alpha)
  V/1 -> Mux/1
  p,q,r/1 -> Mux/3
  Actuators/1 -> Mux/4
  flag/1 -> Mux/5
  Mach/1 -> Terminator2/1
  Interpreted MATLAB Function/1 -> Coeff/1
  Mux/1 -> Interpreted MATLAB Function/1
  Leading Edge Flap/1(delta_lef (deg)) -> Mux/6

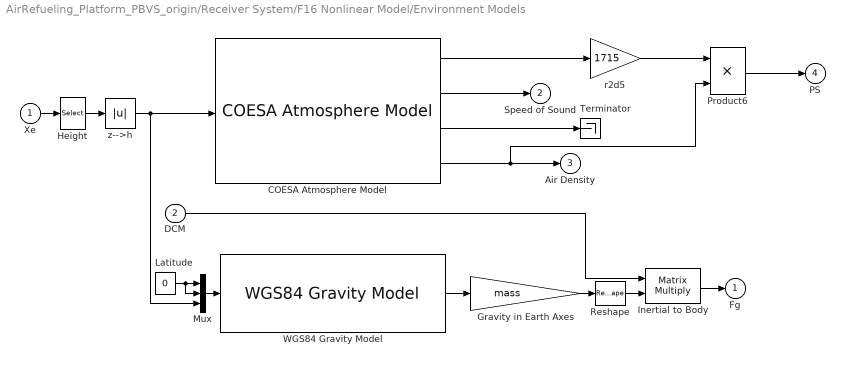
== system AirRefueling_Platform_PBVS_origin/Receiver System/F16 Nonlinear Model/Environment Models ==
  Xe : Inport  PortDimensions=3
  DCM : Inport  Port=2
  COESA Atmosphere Model : aerolibatmos2/COESA Atmosphere Model  units=English (Velocity in ft/s)  spec=1976 COESA-extended U.S. Standard Atmosphere  model=Profile  profile_var=High temperature  profile_percent=10%  profile_alt=5 km (16404 ft)  envelope_var=High temperature  envelope_percent=1%  action=None
  Gravity in Earth Axes : Gain  Gain=mass  SaturateOnIntegerOverflow=on  OutDataTypeStr=Inherit: Same as input  ParamDataTypeStr=Inherit: Same as input
  Height : Selector  InputPortWidth=3  IndexOptions=Index vector (dialog)  Indices=[3]  OutputSizes=1
  Inertial to Body : Product  Multiplication=Matrix(*)  InputSameDT=on  SaturateOnIntegerOverflow=on  OutDataTypeStr=Inherit: Same as first input
  Latitude : Constant  Value=0
  Mux : Mux  Inputs=3
  Product6 : Product  Inputs=**  InputSameDT=on  SaturateOnIntegerOverflow=on  OutDataTypeStr=Inherit: Same as first input
  Reshape : Reshape
  Terminator : Terminator
  "WGS84 Gravity Model " : aerolibobsolete/WGS84 Gravity Model   model=WGS84 Taylor Series  units=English  no_atmos=on  precessing=on  jd_loc=off  month=October  day=10  year=2004  no_centrifugal=on  action=None
  r2d5 : Gain  Gain=1715  SaturateOnIntegerOverflow=on  OutDataTypeStr=Inherit: Same as input  ParamDataTypeStr=Inherit: Same as input
  z-->h : Abs
  Fg : Outport  InitialOutput=0
  Speed of Sound : Outport  Port=2  InitialOutput=0
  Air Density : Outport  Port=3  InitialOutput=0
  PS : Outport  Port=4
  wires:
  Reshape/1 -> Inertial to Body/2
  Mux/1 -> "WGS84 Gravity Model "/1
  z-->h/1 -> Mux/3, COESA Atmosphere Model/1
  COESA Atmosphere Model/2 -> Speed of Sound/1
  COESA Atmosphere Model/3 -> Terminator/1
  Height/1 -> z-->h/1
  Xe/1 -> Height/1
  Latitude/1 -> Mux/2, Mux/1
  "WGS84 Gravity Model "/1 -> Gravity in Earth Axes/1
  Gravity in Earth Axes/1 -> Reshape/1
  DCM/1 -> Inertial to Body/1
  Inertial to Body/1 -> Fg/1
  COESA Atmosphere Model/4 -> Product6/2, Air Density/1
  COESA Atmosphere Model/1 -> r2d5/1
  Product6/1 -> PS/1
  r2d5/1 -> Product6/1

== system AirRefueling_Platform_PBVS_origin/Receiver System/F16 Nonlinear Model/Forces and Moments ==
  Coeff : Inport
  Thrust : Inport  Port=2
  qbar : Inport  Port=3
  "Aerodynamic Forces and Moments " : aerolibadyn/Aerodynamic Forces and Moments   inputAxes=Body  outputForceAxes=Body  outputMomentAxes=Body  S=S_ref  b=b_ref  cbar=d_ref
  Center of Gravity : Constant  Value=[-0 0 0]
  Center of Pressure : Constant  Value=[-0 0 0]
  Sum : Sum  Inputs=++|  InputSameDT=on  SaturateOnIntegerOverflow=on  OutDataTypeStr=Inherit: Same as first input
  X,Y,Z : Outport  InitialOutput=0
  LMN : Outport  Port=2  InitialOutput=0
  wires:
  Center of Pressure/1 -> "Aerodynamic Forces and Moments "/4
  Center of Gravity/1 -> "Aerodynamic Forces and Moments "/3
  "Aerodynamic Forces and Moments "/1 -> Sum/2
  "Aerodynamic Forces and Moments "/2 -> LMN/1
  Sum/1 -> X,Y,Z/1
  Thrust/1 -> Sum/1
  qbar/1 -> "Aerodynamic Forces and Moments "/2
  Coeff/1 -> "Aerodynamic Forces and Moments "/1

== system AirRefueling_Platform_PBVS_origin/Receiver System/F16 Nonlinear Model/actuator ==
  u : Inport
  Aileron Actuator : Subsystem
  Demux : Demux
  Elevator Actuator : Subsystem
  Mux : Mux  Inputs=2
  Mux1 : Mux  Inputs=3
  Mux2 : Mux  Inputs=3
  Rudder Actuator : Subsystem
  Thrust Model : Subsystem
  Ty : Constant  Value=0
  Tz : Constant  Value=0
  Ang : Outport
  T : Outport  Port=2
  uc : Outport  Port=3
  wires:
  u/1 -> Demux/1
  Mux2/1 -> Ang/1, Mux/2
  Thrust Model/1(T) -> Mux/1, Mux1/1  "Tx"
  Ty/1 -> Mux1/2
  Tz/1 -> Mux1/3
  Mux1/1 -> T/1
  Mux/1 -> uc/1
  Demux/1 -> Thrust Model/1(delta_t)
  Elevator Actuator/1(el) -> Mux2/1  "el"
  Aileron Actuator/1(ail) -> Mux2/2  "ail"
  Rudder Actuator/1(rud) -> Mux2/3  "rud"
  Demux/2 -> Elevator Actuator/1(delta_e)
  Demux/3 -> Aileron Actuator/1(delta_a)
  Demux/4 -> Rudder Actuator/1(delta_r)

== system AirRefueling_Platform_PBVS_origin/Receiver System/F16 Nonlinear Model/Aerodynamic Coefficients/Leading Edge Flap ==
  note: see NASA Technical Paper 1538, p34
  note: Initialize LF_state with -alpha0 value in degrees!!!!
  alpha : Inport
  qbar/ps : Inport  Port=2
  Gain : Gain  Gain=2  SaturateOnIntegerOverflow=on  OutDataTypeStr=Inherit: Same as input  ParamDataTypeStr=Inherit: Same as input
  Gain1 : Gain  Gain=7.25  SaturateOnIntegerOverflow=on  OutDataTypeStr=Inherit: Same as input  ParamDataTypeStr=Inherit: Same as input
  Gain2 : Gain  Gain=1.38  SaturateOnIntegerOverflow=on  OutDataTypeStr=Inherit: Same as input  ParamDataTypeStr=Inherit: Same as input
  LEF Actuator : Subsystem
  LF_state : Integrator  InitialCondition=-alpha0
  Sum : Sum  Inputs=-|+|+  InputSameDT=on  SaturateOnIntegerOverflow=on  OutDataTypeStr=Inherit: Same as first input
  Sum1 : Sum  Inputs=|+-  InputSameDT=on  SaturateOnIntegerOverflow=on  OutDataTypeStr=Inherit: Same as first input
  Sum2 : Sum  Inputs=++|  InputSameDT=on  SaturateOnIntegerOverflow=on  OutDataTypeStr=Inherit: Same as first input
  coeff1 : Constant  Value=1.45
  lef Saturation : Saturate  UpperLimit=25  LowerLimit=0
  r2d6 : Gain  Gain=9.05  SaturateOnIntegerOverflow=on  OutDataTypeStr=Inherit: Same as input  ParamDataTypeStr=Inherit: Same as input
  delta_lef (deg) : Outport
  wires:
  Sum1/1 -> Gain1/1
  Gain1/1 -> LF_state/1
  Gain/1 -> Sum2/1
  Gain2/1 -> Sum/2
  coeff1/1 -> Sum/3
  Sum2/1 -> Sum1/2, Gain2/1
  LF_state/1 -> Sum2/2
  alpha/1 -> Sum1/1, Gain/1
  qbar/ps/1 -> r2d6/1
  r2d6/1 -> Sum/1
  lef Saturation/1 -> delta_lef (deg)/1
  Sum/1 -> LEF Actuator/1(dlef)
  LEF Actuator/1(LEF) -> lef Saturation/1

== system AirRefueling_Platform_PBVS_origin/Receiver System/F16 Nonlinear Model/actuator/Aileron Actuator ==
  delta_a : Inport
  Command Saturation : Saturate  UpperLimit=21.5  LowerLimit=-21.5
  Gain : Gain  Gain=20.2  SaturateOnIntegerOverflow=on  OutDataTypeStr=Inherit: Same as input  ParamDataTypeStr=Inherit: Same as input
  "Integrator " : Integrator  InitialCondition=trim_ail  UpperSaturationLimit=21.5  LowerSaturationLimit=-21.5
  Rate Saturation : Saturate  UpperLimit=80  LowerLimit=-80
  Sum : Sum  Inputs=|+-  InputSameDT=on  SaturateOnIntegerOverflow=on  OutDataTypeStr=Inherit: Same as first input
  ail : Outport
  wires:
  delta_a/1 -> Command Saturation/1
  "Integrator "/1 -> ail/1, Sum/2
  Sum/1 -> Gain/1
  Gain/1 -> Rate Saturation/1
  Command Saturation/1 -> Sum/1
  Rate Saturation/1 -> "Integrator "/1

== system AirRefueling_Platform_PBVS_origin/Receiver System/F16 Nonlinear Model/actuator/Elevator Actuator ==
  delta_e : Inport
  Command Saturation : Saturate  UpperLimit=25  LowerLimit=-25
  Gain : Gain  Gain=20.2  SaturateOnIntegerOverflow=on  OutDataTypeStr=Inherit: Same as input  ParamDataTypeStr=Inherit: Same as input
  "Integrator " : Integrator  InitialCondition=trim_ele  UpperSaturationLimit=25  LowerSaturationLimit=-25
  Rate Saturation : Saturate  UpperLimit=60  LowerLimit=-60
  Sum : Sum  Inputs=|+-  InputSameDT=on  SaturateOnIntegerOverflow=on  OutDataTypeStr=Inherit: Same as first input
  el : Outport
  wires:
  delta_e/1 -> Command Saturation/1
  Command Saturation/1 -> Sum/1
  Sum/1 -> Gain/1
  Gain/1 -> Rate Saturation/1
  "Integrator "/1 -> el/1, Sum/2
  Rate Saturation/1 -> "Integrator "/1

== system AirRefueling_Platform_PBVS_origin/Receiver System/F16 Nonlinear Model/actuator/Rudder Actuator ==
  delta_r : Inport
  Command Saturation : Saturate  UpperLimit=30  LowerLimit=-30
  Gain : Gain  Gain=20.2  SaturateOnIntegerOverflow=on  OutDataTypeStr=Inherit: Same as input  ParamDataTypeStr=Inherit: Same as input
  "Integrator " : Integrator  InitialCondition=trim_rud  UpperSaturationLimit=30  LowerSaturationLimit=-30
  Rate Saturation : Saturate  UpperLimit=120  LowerLimit=-120
  Sum : Sum  Inputs=|+-  InputSameDT=on  SaturateOnIntegerOverflow=on  OutDataTypeStr=Inherit: Same as first input
  rud : Outport
  wires:
  "Integrator "/1 -> rud/1, Sum/2
  Sum/1 -> Gain/1
  delta_r/1 -> Command Saturation/1
  Rate Saturation/1 -> "Integrator "/1
  Gain/1 -> Rate Saturation/1
  Command Saturation/1 -> Sum/1

== system AirRefueling_Platform_PBVS_origin/Receiver System/F16 Nonlinear Model/actuator/Thrust Model ==
  delta_t : Inport
  Command Saturation : Saturate  UpperLimit=19000  LowerLimit=1000
  Gain : Gain  SaturateOnIntegerOverflow=on  OutDataTypeStr=Inherit: Same as input  ParamDataTypeStr=Inherit: Same as input
  "Integrator " : Integrator  InitialCondition=trim_thrust  UpperSaturationLimit=30  LowerSaturationLimit=-30
  Rate Saturation : Saturate  UpperLimit=10000  LowerLimit=-10000
  Sum : Sum  Inputs=|+-  InputSameDT=on  SaturateOnIntegerOverflow=on  OutDataTypeStr=Inherit: Same as first input
  T : Outport
  wires:
  delta_t/1 -> Command Saturation/1
  Gain/1 -> Rate Saturation/1
  "Integrator "/1 -> T/1, Sum/2
  Command Saturation/1 -> Sum/1
  Sum/1 -> Gain/1
  Rate Saturation/1 -> "Integrator "/1

== system AirRefueling_Platform_PBVS_origin/Receiver System/F16 Nonlinear Model/Aerodynamic Coefficients/Leading Edge Flap/LEF Actuator ==
  dlef : Inport
  Command Saturation : Saturate  UpperLimit=25  LowerLimit=0
  Gain3 : Gain  Gain=1/0.136  SaturateOnIntegerOverflow=on  OutDataTypeStr=Inherit: Same as input  ParamDataTypeStr=Inherit: Same as input
  "Integrator " : Integrator  InitialCondition=dLEF  UpperSaturationLimit=21.5  LowerSaturationLimit=-21.5
  Rate Saturation : Saturate  UpperLimit=25  LowerLimit=-25
  Sum3 : Sum  Inputs=|+-  InputSameDT=on  SaturateOnIntegerOverflow=on  OutDataTypeStr=Inherit: Same as first input
  LEF : Outport
  wires:
  Gain3/1 -> Rate Saturation/1
  Rate Saturation/1 -> "Integrator "/1
  "Integrator "/1 -> LEF/1, Sum3/2
  Sum3/1 -> Gain3/1
  dlef/1 -> Command Saturation/1
  Command Saturation/1 -> Sum3/1

== matlab function AirRefueling_Platform_PBVS_origin/Visual Servo Block/MATLAB Function3 ==
  data: u1 input; yy output; u2 input; u3 input; t input
function yy = fcn(u1,u2,u3,t)
%#codegen
L=u1;
N=u2;
Ir=u3;
t0=0.25;
%S=zeros(N,2);
dX=zeros(10,1);
dY=zeros(10,1);


 for k=1:N
     [r,c]=find(L == k);
     dX(k)=mean(r);
     dY(k)=mean(c);     
 end
% %plot(S(:,1),S(:,2),'+')
% % dx(:,1)=S(:,1)-mean(S(:,1));
% % dy(:,1)=S(:,2)-mean(S(:,2));
% 
% dX=S(:,1);
% dY=S(:,2);
[mm,nn]=size(Ir);

if N==6
   [dX_up,I]=min(dX(1:6));
   

   
   if t>t0
   aa=dX(I)-mean([dX(1:I);dX(I+1:6)]);
   bb=(max(dY(1:6))-min(dY(1:6)))/6;
   
   if abs(aa/bb)>0.2

       for i=1:6
           if(i~=I)
               for j=1:29
                   i1=floor(dX(I)+(dX(i)-dX(I))/30*j);
                   j1=floor(dY(I)+(dY(i)-dY(I))/30*j);  
                   if(i1>=1&&j1>=1&&i1<=mm&&j1<=nn)              
                       Ir(i1:i1,j1:j1)=1;         
                   end             
               end    
           end       
       end          
   
   end       
       
       

   end
   dX(I:9)=dX(I+1:10); 
   dY(I:9)=dY(I+1:10);    
end

if t>t0+0.05
    ll=4;
    if N==4
       ll=3; 
    end
    if N>6
       ll=4;
    end
    
    for i=1:ll
       for j=1:19
           i1=floor(dX(i)+(dX(i+1)-dX(i))/20*j);
           j1=floor(dY(i)+(dY(i+1)-dY(i))/20*j);  
           if(i1>=1&&j1>=1&&i1<=mm&&j1<=nn)              
               Ir(i1:i1,j1:j1)=1;         
           end             
       end          
    end     
end

% 
% 
% 
% m=[dX(1:N,1) dY(1:N,1) ones(size(dX(1:N,1)))]\-(dX(1:N,1).^2+dY(1:N,1).^2);
% cX=-0.5*m(1);
% cY=-0.5*m(2);
% cR=sqrt((m(1)^2+m(2)^2)/4-m(3));
% 
% 
% %yy=N;
% % 
% %yy = [cX,cY,cR];
% %yy=[yy,N];
% 
% % 
% alpha=0:pi/100:2*pi;
% x=cR*cos(alpha)+cX;
% y=cR*sin(alpha)+cY;
% 
% % if isempty(Ir)
% %     Ir=zeros(720,1280);    
% % end
% 
% [mm,nn]=size(Ir);
% for k=1:length(alpha)
% 
%     i=floor(x(k));
%     j=floor(y(k));
%     if(i>=1&&j>=1&&i+1<=mm&&j+1<=nn)
%         Ir(i:i+1,j:j+1)=1;        
%     end
%         
% end
% 
% i=floor(cX);
% j=floor(cY);
% 
% if(i-3>=1&&j-3>=1&&i+4<=mm&&j+4<=nn)
%     Ir(i-3:i+4,j:j+1)=1; 
%     Ir(i:i+1,j-3:j+4)=1;  
% end
% 
% % 
% 
% 
% 
yy=Ir;

== matlab function AirRefueling_Platform_PBVS_origin/Visual Servo Block/MATLAB Function4 ==
  data: u1 input; y output; u2 input
function y = fcn(u1,u2)
%#codegen

%y = u1;
y = u1+u2;

== matlab function AirRefueling_Platform_PBVS_origin/Hose-Drogue System/HDU Function ==
  data: t input; u input; y3 output; dp input
function y3  = fcn(t,u,dp)
% persistent hwpState;
% if isempty(hwpState)
%     hwpState=zeros(20,1);
% end

ll=zeros(20,1);
for i=1:20
    if i==1
       uk_1 = [0;0;0];
    else
        uk_1 = [u(3*(i-1)-2);u(3*(i-1)-2+1);u(3*(i-1)-2+2)];
    end
    uk = [u(3*(i)-2);u(3*(i)-2+1);u(3*(i)-2+2)];
    
    ll(i)=sqrt((uk(1)-uk_1(1))^2+(uk(2)-uk_1(2))^2+(uk(3)-uk_1(3))^2);
end

y = sum(ll);

y1= sqrt((u(58))^2+(u(59))^2+(u(60))^2);
y2 = y1-y;

y3  = 0;

% hwpState = [((y1/14.29*14.33-y)/y);hwpState(1:19)];

% rolldown = true;
% for i=1:20
%     if hwpState(i)<-0.0005
%         rolldown =false;
%         break;
%     end
% end

rolldown = false;
if dp(1)<-0.3 && ((y1/14.29*14.33-y)/y) >=-0.001
    rolldown = true;
end

if rolldown
    y3=sat((y-14.33)/1)*1*1.2;
else
    y3=0;
    if ((y1/14.29*14.33-y)/y) <=-0.01
        y3 = -4*(y1/14.29*14.33-y);
    elseif ((y1/14.29*14.33-y)/y) <=-0.0015
        y3 = -2*(y1/14.29*14.33-y);
%     elseif((y1/14.29*14.33-y)/y) <=-0.0015
%         y3 = -3*(y1/14.29*14.33-y);
    end    
end




% elseif ((y1/14.29*14.33-y)/y) >=-0.001
%     y3=sat((y-14.33)/0.8)*0.8*0.8;
% end


if t<12
    y3=0;
end

y2=(y1/14.29*14.33-y)/y;

== matlab function AirRefueling_Platform_PBVS_origin/Hose-Drogue System/Subsystem/MATLAB Function ==
  data: u input; y output
function y = fcn(u)
y=0;

if u<=3
    y=14;
end
if u<=13 && u>3
    y=14-((u-3)*14/10);
end

== matlab function AirRefueling_Platform_PBVS_origin/Hose-Drogue System/Collision Model ==
  settings: updateMethod=DISCRETE
  data: u input; y output; v input
function y = fcn(u,v)

u(1) = u(1)-0.1; % Redefine the drogue center.

persistent isXCrossBound;
if isempty(isXCrossBound)
    isXCrossBound = false;
end

persistent isRCrossBound;
if isempty(isRCrossBound)
    isRCrossBound = false;
end


persistent lastPosState;
if isempty(lastPosState)
    lastPosState = [0;0;0];
end


if ~isXCrossBound && lastPosState(1)<=0 && u(1)>0
    isXCrossBound =true;
end

if isXCrossBound&& u(1)<-0.05 && lastPosState(1) >= -0.05
    isXCrossBound=false;
end


R = sqrt(u(2)^2+u(3)^2);
RLast = sqrt(lastPosState(2)^2+lastPosState(3)^2);

RDrogue = 0.2;
 if u(1)>-0.15 && u(1)<0
     RDrogue = 0.1*(-u(1)/0.15)+0.1;
 end
 
 if u(1)>=0
     RDrogue = 0.1;
 end


if ~isRCrossBound &&  R>(RDrogue+0.015) && u(1)>-0.1 && (u(1)<=0 || isXCrossBound) && RLast <=(RDrogue+0.01)
    isRCrossBound = true;
end

if isRCrossBound  && R<RDrogue && u(1)>-0.15 && (u(1)<=0 || isXCrossBound) && RLast>=RDrogue
    isRCrossBound = false;
end

if isRCrossBound && u(1)<=-0.15 && ~isXCrossBound
    isRCrossBound = false;
end


y=[0;0;0];


if isXCrossBound
    if u(1) <0.05
        y(1)=2000*u(1);
        if v(1)>0
            y(1) = y(1) + 1000*v(1);
            y(2)=600*v(2);
            y(3)=600*v(3);
        end  
    else
         y(1) = 1000*u(1)+3000*v(1);
         y(2)=200*v(2);
         y(3)=200*v(3);         
    end 
end

eR = R - RDrogue;
if ~isXCrossBound && u(1)>-0.1 && u(1)<=0.1 && eR<=0 
      y(2)=200*v(2);
      y(3)=200*v(3); 
end


if isRCrossBound
    if eR < 0.05
        Ru = 5000*eR;
        y(2) = Ru*u(2)/R;
        y(3) = Ru*u(3)/R;
        if R>RLast
            y(2) = y(2)+ 200*v(2);
            y(3) = y(3)+ 200*v(3);
        end
    else
            Ru = 10000*eR;
            y(2) = Ru*u(2)/R+50*v(2);
            y(3) = Ru*u(3)/R+50*v(3);              
    end
end

lastPosState = u;


%y=[0;0;0];
% if u(1)<-0.1 && (u(2) > 0.05)

% if u(1)>0 && v(1)>0
% %     if v(1)>=1
% %         y(1)=1000*v(1);
% %         if(u(1)>0.05)
% %             y(1)= y(1)+10000*u(1);
% %         end
% %     else
% %         if(u(1)>0.05)
% %             y(1)=10000*u(1);
% %         else
% %             y(1)=500*u(1)+100*v(1);
% %         end 
% %     end
%     y(1)=1000*u(1);
%     if u(1)>0.01
%         y(1)=2000*u(1);
%     end
%     
%     if u(1)>0.02
%         y(1)=5000*u(1);
%     end  
%     %y(1)=y(1)+100*v(1);
%     
% end


% if u(1)>-0.1 && u(2) > 0.05 %&& u(2) <0.08
%     y(2)=5000*(u(2)-0.05);
% end
% 
% if u(1)>-0.1 && u(2) <- 0.05 %&&  u(2) >- 0.08
%     y(2)=5000*(u(2)+0.05);
% end
% 
% if u(1)>-0.1 && u(3) > 0.05 %&&  u(3) < 0.08
%     y(3)=5000*(u(3)-0.05);
% end
% 
% if u(1)>-0.1 && u(3) <- 0.05 %&& u(3) >- 0.08
%     y(3)=5000*(u(3)+0.05);
% end




% if u(1)>-0.15 && u(3) > 0.2
%     if v(3)>=1
%         y(3)=1000*v(3);
%     else
%         y(3)=5000*(u(3)-0.2)+100*v(3);
%     end
% end
% 
% if u(1)>-0.15 && u(3) <- 0.2
%     if v(3)<=-1
%         y(3)=1000*v(3);
%     else
%         y(3)=5000*(u(3)+0.2)+100*v(3);
%     end
% end

== matlab function AirRefueling_Platform_PBVS_origin/Tanker System/  ==
  data: u input; y output

function y = WindTurFromTank(u)
%#codegen

%横纵向气流角速度等下计算长度
c_lat=4;
c_lon=4;

%两端参考点
u1 = u+[0 ,c_lat ,0]';
u2 = u+[0 ,-c_lat, 0]';

yy1 = TankerVortexWindField(u1);
yy2 = TankerVortexWindField(u2);

%计算x轴向滚转角速度
yp = (yy1(3) - yy2(3))/4/c_lat;

u3=u+[c_lon, 0,0]';
u4=u+[-c_lon ,0,0]';
yy3 = TankerVortexWindField(u3);
yy4 = TankerVortexWindField(u4);

%俯仰角速度计算
yq = -(yy3(3) - yy4(3))/4/c_lon;

%偏航角速度设为0
yr = 0;

%质心处风场计算
y_uvw = TankerVortexWindField(u);


%y = [y_uvw(1);y_uvw(2);y_uvw(3);-yp;-yq;-yr]*0.5;
y = [y_uvw(1);y_uvw(2);y_uvw(3);-yp;-yq;-yr];
